simulink model "outerControllerTuning"  (R2018a)
settings: Solver=VariableStepAuto  StartTime=0.0  StopTime=50.0  RelTol=1e-3
values from neighbouring files (symbols this model uses):
  d = 2.4*10^-3    (= 0.0024)    [innerInit.m]    (also in outerInit.m)
  g = 9.81    [innerInit.m]    (also in outerInit.m)
  Ixx = 5.9*10-3    (= 56)    [innerInit.m]    (also in outerInit.m = 0.0059)
  Iyy = 5.9*10-3    (= 56)    [innerInit.m]    (also in outerInit.m = 0.0059)
  Izz = 1.16*10-3    (= 8.6)    [innerInit.m]    (also in outerInit.m = 0.00116)
  kr = 1/2    (= 0.5)    [innerInit.m]    (also in outerInit.m = 0.1)
  kt = 1/2    (= 0.5)    [innerInit.m]    (also in outerInit.m = 0.1)
  l = 0.255    [innerInit.m]    (also in outerInit.m)
  m = 0.5    [innerInit.m]    (also in outerInit.m)
libraries: simulink x4
settings Model: Creator=dinies33  LastModifiedBy=blue_orangotan

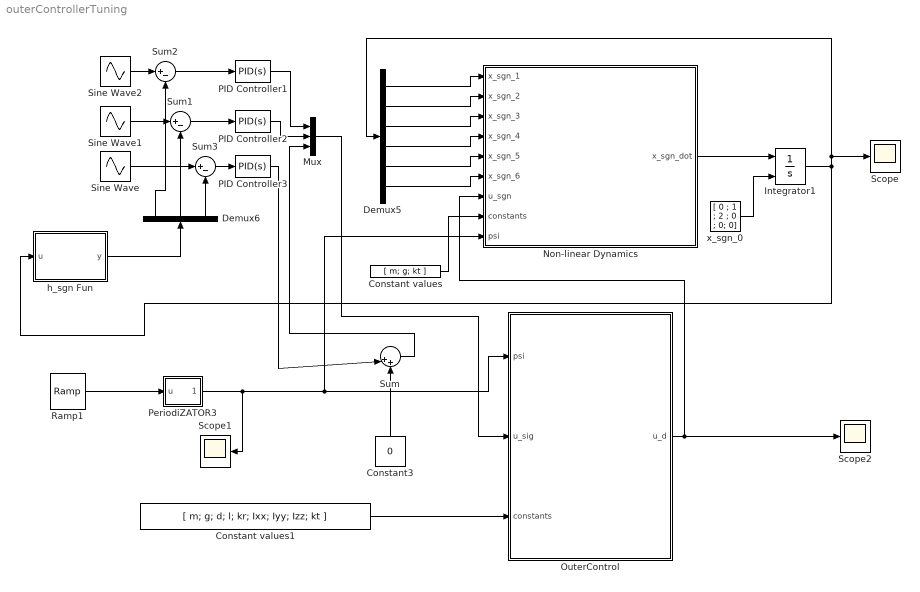
== system outerControllerTuning ==
  Constant values : Constant  Value=[ m; g; kt ]
  Constant values1 : Constant  Value=[ m; g; d; l; kr; Ixx; Iyy; Izz; kt ]
  Constant3 : Constant  Value=0
  Demux5 : Demux  Outputs=6
  Demux6 : Demux  Outputs=3
  Integrator1 : Integrator  InitialConditionSource=external
  Mux : Mux  Inputs=3
  Non-linear Dynamics : MATLAB Function  TreatAsAtomicUnit=on
  OuterControl : MATLAB Function  TreatAsAtomicUnit=on
  PID Controller1 : simulink/Continuous/PID Controller  Controller=PID  TimeDomain=Continuous-time  SampleTime=-1  IntegratorMethod=Forward Euler  FilterMethod=Forward Euler  Form=Parallel  UseFilter=on  ControllerParametersSource=internal  P=0.939601981976548  I=0.0298455660718895  D=4.45438528962657  N=508.848592355901  InitialConditionSource=internal  InitialConditionForIntegrator=0  InitialConditionForFilter=0  ExternalReset=none  LimitOutput=off  UpperSaturationLimit=inf  LowerSaturationLimit=-inf  LinearizeAsGain=on  AntiWindupMode=none  Kb=1  TrackingMode=off  Kt=1  PParamMin=[]  PParamMax=[]  IParamMin=[]  IParamMax=[]  DParamMin=[]  DParamMax=[]  NParamMin=[]  NParamMax=[]  KbParamMin=[]  KbParamMax=[]  KtParamMin=[]  KtParamMax=[]  POutMin=[]  POutMax=[]  IOutMin=[]  IOutMax=[]  DOutMin=[]  DOutMax=[]  NOutMin=[]  NOutMax=[]  KbOutMin=[]  KbOutMax=[]  KtOutMin=[]  KtOutMax=[]  IntegratorOutMin=[]  IntegratorOutMax=[]  FilterOutMin=[]  FilterOutMax=[]  SumOutMin=[]  SumOutMax=[]  SumI1OutMin=[]  SumI1OutMax=[]  SumI2OutMin=[]  SumI2OutMax=[]  SumI3OutMin=[]  SumI3OutMax=[]  SumDOutMin=[]  SumDOutMax=[]  SaturationOutMin=[]  SaturationOutMax=[]  IntegratorContinuousStateAttributes=''  IntegratorStateMustResolveToSignalObject=off  IntegratorRTWStateStorageClass=Auto  FilterContinuousStateAttributes=''  FilterStateMustResolveToSignalObject=off  FilterRTWStateStorageClass=Auto  DifferentiatorICPrevScaledInput=0  DifferentiatorOutMin=[]  DifferentiatorOutMax=[]  FilterDiffOutCoefMin=[]  FilterDiffOutCoefMax=[]  SumDenOutMin=[]  SumDenOutMax=[]  SumNumOutMin=[]  SumNumOutMax=[]  ReciprocalOutMin=[]  ReciprocalOutMax=[]  DivideOutMin=[]  DivideOutMax=[]  TunerSelectOption=Transfer Function Based (PID Tuner App)
  PID Controller2 : simulink/Continuous/PID Controller  Controller=PID  TimeDomain=Continuous-time  SampleTime=-1  IntegratorMethod=Forward Euler  FilterMethod=Forward Euler  Form=Parallel  UseFilter=on  ControllerParametersSource=internal  P=0.942155734377191  I=0.0299673249963071  D=4.46043448837536  N=509.539625142761  InitialConditionSource=internal  InitialConditionForIntegrator=0  InitialConditionForFilter=0  ExternalReset=none  LimitOutput=off  UpperSaturationLimit=inf  LowerSaturationLimit=-inf  LinearizeAsGain=on  AntiWindupMode=none  Kb=1  TrackingMode=off  Kt=1  PParamMin=[]  PParamMax=[]  IParamMin=[]  IParamMax=[]  DParamMin=[]  DParamMax=[]  NParamMin=[]  NParamMax=[]  KbParamMin=[]  KbParamMax=[]  KtParamMin=[]  KtParamMax=[]  POutMin=[]  POutMax=[]  IOutMin=[]  IOutMax=[]  DOutMin=[]  DOutMax=[]  NOutMin=[]  NOutMax=[]  KbOutMin=[]  KbOutMax=[]  KtOutMin=[]  KtOutMax=[]  IntegratorOutMin=[]  IntegratorOutMax=[]  FilterOutMin=[]  FilterOutMax=[]  SumOutMin=[]  SumOutMax=[]  SumI1OutMin=[]  SumI1OutMax=[]  SumI2OutMin=[]  SumI2OutMax=[]  SumI3OutMin=[]  SumI3OutMax=[]  SumDOutMin=[]  SumDOutMax=[]  SaturationOutMin=[]  SaturationOutMax=[]  IntegratorContinuousStateAttributes=''  IntegratorStateMustResolveToSignalObject=off  IntegratorRTWStateStorageClass=Auto  FilterContinuousStateAttributes=''  FilterStateMustResolveToSignalObject=off  FilterRTWStateStorageClass=Auto  DifferentiatorICPrevScaledInput=0  DifferentiatorOutMin=[]  DifferentiatorOutMax=[]  FilterDiffOutCoefMin=[]  FilterDiffOutCoefMax=[]  SumDenOutMin=[]  SumDenOutMax=[]  SumNumOutMin=[]  SumNumOutMax=[]  ReciprocalOutMin=[]  ReciprocalOutMax=[]  DivideOutMin=[]  DivideOutMax=[]  TunerSelectOption=Transfer Function Based (PID Tuner App)
  PID Controller3 : simulink/Continuous/PID Controller  Controller=PID  TimeDomain=Continuous-time  SampleTime=-1  IntegratorMethod=Forward Euler  FilterMethod=Forward Euler  Form=Parallel  UseFilter=on  ControllerParametersSource=internal  P=0.939353785780563  I=0.0298337412778135  D=4.45379693701357  N=508.781381652965  InitialConditionSource=internal  InitialConditionForIntegrator=0  InitialConditionForFilter=0  ExternalReset=none  LimitOutput=off  UpperSaturationLimit=inf  LowerSaturationLimit=-inf  LinearizeAsGain=on  AntiWindupMode=none  Kb=1  TrackingMode=off  Kt=1  PParamMin=[]  PParamMax=[]  IParamMin=[]  IParamMax=[]  DParamMin=[]  DParamMax=[]  NParamMin=[]  NParamMax=[]  KbParamMin=[]  KbParamMax=[]  KtParamMin=[]  KtParamMax=[]  POutMin=[]  POutMax=[]  IOutMin=[]  IOutMax=[]  DOutMin=[]  DOutMax=[]  NOutMin=[]  NOutMax=[]  KbOutMin=[]  KbOutMax=[]  KtOutMin=[]  KtOutMax=[]  IntegratorOutMin=[]  IntegratorOutMax=[]  FilterOutMin=[]  FilterOutMax=[]  SumOutMin=[]  SumOutMax=[]  SumI1OutMin=[]  SumI1OutMax=[]  SumI2OutMin=[]  SumI2OutMax=[]  SumI3OutMin=[]  SumI3OutMax=[]  SumDOutMin=[]  SumDOutMax=[]  SaturationOutMin=[]  SaturationOutMax=[]  IntegratorContinuousStateAttributes=''  IntegratorStateMustResolveToSignalObject=off  IntegratorRTWStateStorageClass=Auto  FilterContinuousStateAttributes=''  FilterStateMustResolveToSignalObject=off  FilterRTWStateStorageClass=Auto  DifferentiatorICPrevScaledInput=0  DifferentiatorOutMin=[]  DifferentiatorOutMax=[]  FilterDiffOutCoefMin=[]  FilterDiffOutCoefMax=[]  SumDenOutMin=[]  SumDenOutMax=[]  SumNumOutMin=[]  SumNumOutMax=[]  ReciprocalOutMin=[]  ReciprocalOutMax=[]  DivideOutMin=[]  DivideOutMax=[]  TunerSelectOption=Transfer Function Based (PID Tuner App)
  PeriodiZATOR3 : MATLAB Function  TreatAsAtomicUnit=on
  Ramp1 : simulink/Sources/Ramp  slope=0.3  start=0  InitialOutput=0
  Scope : Scope
  Scope1 : Scope
  Scope2 : Scope
  Sine Wave : Sin  SampleTime=0
  Sine Wave1 : Sin  SampleTime=0
  Sine Wave2 : Sin  SampleTime=0
  Sum : Sum  Inputs=||++
  Sum1 : Sum  Inputs=|+-
  Sum2 : Sum  Inputs=|+-
  Sum3 : Sum  Inputs=|+-
  h_sgn Fun : MATLAB Function  TreatAsAtomicUnit=on
  x_sgn_0 : Constant  Value=[ 0 ; 1 ; 2 ; 0 ; 0; 0]
  wires:
  Constant values/1 -> Non-linear Dynamics/8(constants)
  Non-linear Dynamics/1(x_sgn_dot) -> Integrator1/1
  Integrator1/1 -> Scope/1, Demux5/1, h_sgn Fun/1(u)
  x_sgn_0/1 -> Integrator1/2
  Demux5/1 -> Non-linear Dynamics/1(x_sgn_1)
  Demux5/2 -> Non-linear Dynamics/2(x_sgn_2)
  Demux5/3 -> Non-linear Dynamics/3(x_sgn_3)
  Demux5/4 -> Non-linear Dynamics/4(x_sgn_4)
  Demux5/5 -> Non-linear Dynamics/5(x_sgn_5)
  Demux5/6 -> Non-linear Dynamics/6(x_sgn_6)
  Demux6/1 -> Sum2/2
  Demux6/2 -> Sum1/2
  h_sgn Fun/1(y) -> Demux6/1
  Sine Wave/1 -> Sum3/1
  Sum3/1 -> PID Controller3/1
  Sum1/1 -> PID Controller2/1
  Sine Wave2/1 -> Sum2/1
  Sine Wave1/1 -> Sum1/1
  Sum2/1 -> PID Controller1/1
  Demux6/3 -> Sum3/2
  PID Controller1/1 -> Mux/1
  PID Controller2/1 -> Mux/2
  PID Controller3/1 -> Sum/1
  Sum/1 -> Mux/3
  Constant3/1 -> Sum/2
  Ramp1/1 -> PeriodiZATOR3/1(u)
  PeriodiZATOR3/1(angle) -> Scope1/1, Non-linear Dynamics/9(psi), OuterControl/1(psi)
  Constant values1/1 -> OuterControl/3(constants)
  Mux/1 -> OuterControl/2(u_sig)
  OuterControl/1(u_d) -> Non-linear Dynamics/7(u_sgn), Scope2/1

== matlab function outerControllerTuning/h_sgn Fun ==
  data: u input; y output
function y = fcn(u)

h = [
    1 0 0 0 0 0;
    0 1 0 0 0 0;
    0 0 1 0 0 0;
    ];
    
y = h*u;

== matlab function outerControllerTuning/Non-linear Dynamics ==
  data: x_sgn_1 input; x_sgn_dot output; x_sgn_2 input; x_sgn_3 input; x_sgn_4 input; x_sgn_5 input; x_sgn_6 input; u_sgn input; constants input; psi input
function x_sgn_dot = fcn(x_sgn_1,x_sgn_2,x_sgn_3,x_sgn_4,x_sgn_5,x_sgn_6,u_sgn,constants, psi)
 
m= constants(1,1);
g= constants(2,1);
kt = constants(3,1);
 
% x_sgn = [x_sgn_1;
%         x_sgn_2;
%         x_sgn_3;
%         x_sgn_4;
%         x_sgn_5;
%         x_sgn_6];
    
% A = zeros(6);
% A(1:3,4:6) = eye(3);
% A(4:6,4:6) = -kt*m*eye(3);
% 
% G= zeros(6,3);
% G(4:6,:) = eye(3);

f = [x_sgn_4; 
     x_sgn_5;
     x_sgn_6;
     cos(psi)*u_sgn(2) + sin(psi)*u_sgn(1) - kt/m*x_sgn_4;
     sin(psi)*u_sgn(2) - cos(psi)*u_sgn(1) - kt/m*x_sgn_5;
     u_sgn(3) - kt/m*x_sgn_6 - g];


% x_sgn_dot = A*x_sgn + G*u_sgn_sgn + [ 0 0 0 0 0 -g]' ;
x_sgn_dot = f;

== matlab function outerControllerTuning/OuterControl ==
  data: psi input; u_d output; u_sig input; constants input
function u_d = fcn(psi, u_sig, constants)

m= constants(1,1);
d= constants(3,1);
kr= constants(5,1);

u1_sig_sig = u_sig(1);
u2_sig_sig = u_sig(2);
u3_sig = u_sig(3);

R = [sin(psi), cos(psi);
    -cos(psi), sin(psi)];

u_sig_sig = [u1_sig_sig u2_sig_sig]';

u12 = R'*u_sig_sig;

u_d = [0 0 0]';
u_d(1) = u12(1);
u_d(2)= u12(2);
u_d(3) = u3_sig+9.81;

== matlab function outerControllerTuning/PeriodiZATOR3 ==
  data: u input; angle output
function angle = fcn(u)

y = sin(u);
x = cos(u);

% angle = mod(u, 2*pi);
angle = atan2(y,x);
